simulink model "testPID_SteadyRotation"  (R2021a)
settings: Solver=VariableStepAuto  StartTime=0.0  StopTime=Torb  RelTol=1e-3
values from neighbouring files (symbols this model uses):
  Tmax = Fmax*Larm    (= 0.00125)    [control_1.m]    (also in control_2.m; control_3.m; control_4.m; control_extra2.m)
  wz_desired = 20*pi/Torb    [control_3.m]    (also in control_4.m)
libraries: simulink x1, sharedtransform x1
settings Model: DataDictionary=databus.sldd  Creator=Laura  LastModifiedBy=Laura

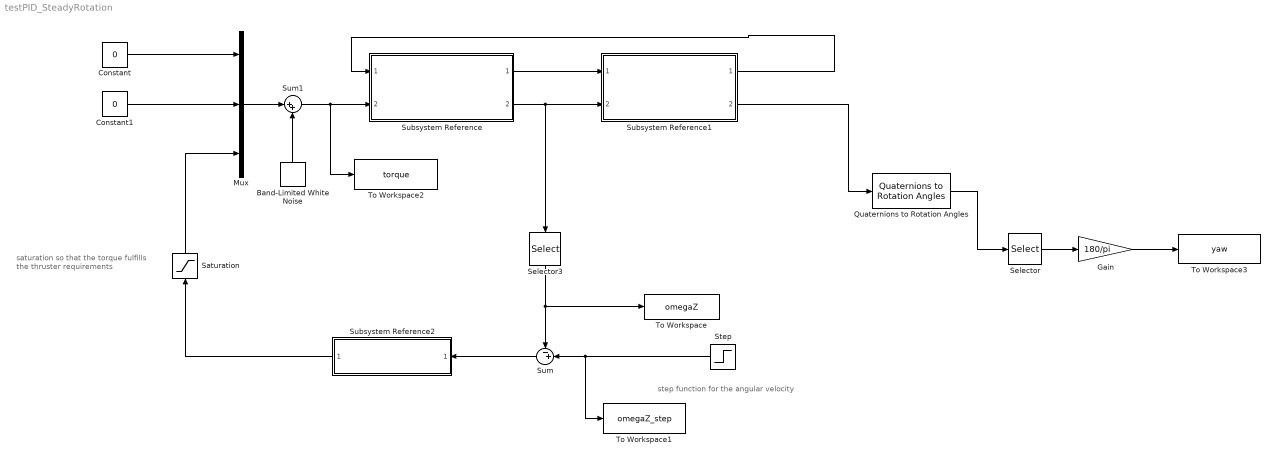
== system testPID_SteadyRotation ==
  note: step function for the angular velocity
  note: saturation so that the torque fulfills the thruster requirements
  Band-Limited White Noise : simulink/Sources/Band-Limited White Noise  Cov=[1e-12]  Ts=0.1  seed=[23341]
  Constant : Constant  Value=0
  Constant1 : Constant  Value=0
  Gain : Gain  Gain=180/pi
  Mux : Mux  Inputs=3
  Quaternions to Rotation Angles : sharedtransform/Quaternions to Rotation Angles  rotationOrder=ZYX  aMode=aMode
      settings: SourceProductBaseCode=AE,PW,DR,MT,UV,VE
  Saturation : Saturate  UpperLimit=Tmax  LowerLimit=-Tmax
  Selector : Selector  InputPortWidth=3  IndexOptions=Index vector (dialog)  Indices=[1]  OutputSizes=1
  Selector3 : Selector  InputPortWidth=3  IndexOptions=Index vector (dialog)  Indices=[3]  OutputSizes=1
  Step : Step  Time=0  After=wz_desired  SampleTime=0
  Subsystem Reference : Subsystem  ReferencedSubsystem=Dynamics
  Subsystem Reference1 : Subsystem  ReferencedSubsystem=Kinematics
  Subsystem Reference2 : Subsystem  ReferencedSubsystem=PID
  Sum : Sum  Inputs=-+|
  Sum1 : Sum  Inputs=|++
  To Workspace : ToWorkspace  VariableName=omegaZ  SaveFormat=Timeseries  SampleTime=-1
  To Workspace1 : ToWorkspace  VariableName=omegaZ_step  SaveFormat=Timeseries  SampleTime=-1
  To Workspace2 : ToWorkspace  VariableName=torque  SaveFormat=Timeseries  SampleTime=-1
  To Workspace3 : ToWorkspace  VariableName=yaw  SaveFormat=Timeseries  SampleTime=-1
  wires:
  Subsystem Reference1/1 -> Subsystem Reference/1
  Subsystem Reference1/2 -> Quaternions to Rotation Angles/1
  Subsystem Reference/2 -> Selector3/1, Subsystem Reference1/2
  Subsystem Reference/1 -> Subsystem Reference1/1
  Constant/1 -> Mux/1
  Constant1/1 -> Mux/2
  Subsystem Reference2/1 -> Saturation/1
  Quaternions to Rotation Angles/1 -> Selector/1
  Selector/1 -> Gain/1
  Sum/1 -> Subsystem Reference2/1
  Step/1 -> To Workspace1/1, Sum/2
  Selector3/1 -> Sum/1, To Workspace/1
  Band-Limited White Noise/1 -> Sum1/2
  Mux/1 -> Sum1/1
  Sum1/1 -> To Workspace2/1, Subsystem Reference/2
  Saturation/1 -> Mux/3
  Gain/1 -> To Workspace3/1
